simulink model "PubIfDecisionLSM_MDL"  (R2020b)
settings: configuration reference "DspaceConfig" (kept outside this file)
PostLoadFcn:
  | if any(exist('dsrtsu_mdlpostloadfcn', 'file') ~= 0), dsrtsu_mdlpostloadfcn('Execute', bdroot); end
InitFcn:
  | , if any(exist('rtifpga_mdlclblib', 'file') ~= 0), rtifpga_mdlclblib('Init', bdroot); end,
  | , if any(exist('dsmpb_private', 'file') ~= 0), dsmpb_private('dsmpb_mdlclblib', 'Init', bdroot); end,
values from neighbouring files (symbols this model uses):
  P_LSM_ALC_Enable = 0.0    [LSM_Parameter.sldd]
  P_LSM_AwayEdge_offset = 0.1    [LSM_Parameter.sldd]
  P_LSM_CentValidErr = 1.0    [LSM_Parameter.sldd]
  P_LSM_DOP_C0_EN_Limit = 0.8    [LSM_Parameter.sldd]
  P_LSM_DOP_C0_out_Limit = 2.0    [LSM_Parameter.sldd]
  P_LSM_DOP_C1_EN_Limit : value not decoded    [LSM_Parameter.sldd]
  P_LSM_DOP_C1_out_Limit : value not decoded    [LSM_Parameter.sldd]
  P_LSM_DOP_C1AndC2_Lim_X : value not decoded    [LSM_Parameter.sldd]
  P_LSM_DOP_C2_EN_Limit : value not decoded    [LSM_Parameter.sldd]
  P_LSM_DOP_C2_out_Limit : value not decoded    [LSM_Parameter.sldd]
  P_LSM_DOP_In_Pre2Dop_Dis = 1.0    [LSM_Parameter.sldd]
  P_LSM_DOP_Out_Pre2Dop_Dis = 2.0    [LSM_Parameter.sldd]
  P_LSM_DOP_PreDis_X : value not decoded    [LSM_Parameter.sldd]
  P_LSM_DOP_PreDis_Y : value not decoded    [LSM_Parameter.sldd]
  P_LSM_DOPEnableSW = 1.0    [LSM_Parameter.sldd]
  P_LSM_DOPValid_CheckTime = 0.06    [LSM_Parameter.sldd]
  P_LSM_DoubleLine_Curr2Cent_Dislimit = 0.5    [LSM_Parameter.sldd]
  P_LSM_DoubleLine_Dop2Cent_Dislimit = 0.5    [LSM_Parameter.sldd]
  P_LSM_DoubleLine_DOPOut_C1 : value not decoded    [LSM_Parameter.sldd]
  P_LSM_DoubleLine_Pre2Cent_Dislimit = 1.0    [LSM_Parameter.sldd]
  P_LSM_Error_Limit = 0.5    [LSM_Parameter.sldd]
  P_LSM_IFV2CenterAxis = 0.0    [LSM_Parameter.sldd]
  P_LSM_IFV2RearAxis = 0.0    [LSM_Parameter.sldd]
  P_LSM_Line2Edge_limit = 0.5    [LSM_Parameter.sldd]
  P_LSM_Line_Error = 0.1    [LSM_Parameter.sldd]
  P_LSM_LineSTD_Limit = 0.15    [LSM_Parameter.sldd]
  P_LSM_NOH_Switch = 0.0    [LSM_Parameter.sldd]
  P_LSM_OTL_C0_Factor = 1.0    [LSM_Parameter.sldd]
  P_LSM_OTL_C1_Factor = 0.5    [LSM_Parameter.sldd]
  P_LSM_OTL_C2_Factor = 0.5    [LSM_Parameter.sldd]
  P_LSM_Pre2OnlyLineDis = 5.0    [LSM_Parameter.sldd]
  P_LSM_Pre_t = 0.0    [LSM_Parameter.sldd]
  P_LSM_SingleLine_Cent2Edge_Dislimit = 100.0    [LSM_Parameter.sldd]
  P_LSM_SingleLine_Curr2Cent_Dislimit = 0.2    [LSM_Parameter.sldd]
  P_LSM_SingleLine_Dop2Cent_Dislimit = 0.2    [LSM_Parameter.sldd]
  P_LSM_SingleLine_DOPOut_C1 : value not decoded    [LSM_Parameter.sldd]
  P_LSM_SingleLine_Pre2Cent_Dislimit = 0.5    [LSM_Parameter.sldd]
  P_LSM_TJALimitSpd = 60.0    [LSM_Parameter.sldd]
undefined symbols (not defined in the file or in its folder): P_lCS_IFV2CenterAxis, P_LCS_IFV2RearAxis, P_LSM_EntryEdge_offset, P_LSM_EntryLnChngEnSwitch, P_LSM_EntryVanishDis, P_LSM_LinetLostTime, P_LSM_LineWijCal_C12, P_LSM_LineWijCal_C13, P_LSM_MapValid_ErrorSwitch, P_LSM_PosLineLcFac, P_LSM_SpdLim_Stub_Spd, P_LSM_SpdLim_StubLength, P_LSM_SpdTurnAlarm
libraries: simulink x324, TrueDurationTime x11
(part 20 of 25)

== matlab function PubIfDecisionLSM_MDL/Subsystem1/TargetLineCalc_20ms2/TargetLineCalc/HWALineCalc ==
  data: LeftLineTypeEn input boolean size=1; RightLineTypeEn input boolean size=1; YBranch_b input boolean size=1; YBranchRi_b input boolean size=1; HWALineC0K1 input; TJA_Line_State input; HWALineValid output boolean size=1; HWASts input uint8 size=1; HWAStsK1 input uint8 size=1; LineConf input uint8 size=4; Reliable input; A3 input single size=4; A2 input single size=4; A1 input single size=4; A0 input single size=4; Range input single size=4; tLost input single size=4; PathPredValid input boolean size=1; PathPredA3 input single size=1; PathPredA2 input single size=1; PathPredA1 input single size=1; PathPredA0 input single size=1; PathPredRange input; LeftOffset_b input boolean size=1; RightOffset_b input boolean size=1; HWALineC3 output single size=1; HWALineC2 output single size=1; HWALineC1 output single size=1; HWALineC0 output single size=1; HWARange output single size=1; RoadWidth input single size=1; dDeltaX input single size=1; dDeltaY input single size=1; CosOfPsi input single size=1; SinOfPsi input single size=1; vRef input single size=1; DistanceLim input single size=1; HWALeLineValid output boolean size=1; HWALeLineC3 output single size=1; HWALeLineC2 output single size=1; HWALeLineC1 output single size=1; HWALeLineC0 output single size=1; HWALeRange output single size=1; HWARiLineValid output boolean size=1; HWARiLineC3 output single size=1; HWARiLineC2 output single size=1; HWARiLineC1 output single size=1; HWARiLineC0 output single size=1; HWARiRange output single size=1; preDyDiff output single size=1; HeadAngDiff output single size=1; Error output boolean size=1; SingleLineLost_b output boolean size=1; DoubleLineLost_b output boolean size=1; MoveIDK1 input int8 size=1; LockIDK1 input int8; MoveID output int8 size=1; LockID output int8; Lock_counterK1 input uint8; Lock_counter output uint8
function [HWALineValid,HWALineC3,HWALineC2,HWALineC1,HWALineC0,HWARange,...
    HWALeLineValid,HWALeLineC3,HWALeLineC2,HWALeLineC1,HWALeLineC0,HWALeRange,...
    HWARiLineValid,HWARiLineC3,HWARiLineC2,HWARiLineC1,HWARiLineC0,HWARiRange,...
    preDyDiff,HeadAngDiff,Error,SingleLineLost_b,DoubleLineLost_b,MoveID,LockID,Lock_counter] = ...
    LineCalc(LeftLineTypeEn,RightLineTypeEn,YBranch_b,YBranchRi_b,HWALineC0K1,TJA_Line_State,HWASts,HWAStsK1,LineConf,Reliable,A3,A2,A1,A0,Range,tLost,...
    PathPredValid,PathPredA3,PathPredA2,PathPredA1,PathPredA0,PathPredRange,...
    LeftOffset_b,RightOffset_b,RoadWidth,dDeltaX,dDeltaY,CosOfPsi,SinOfPsi,vRef,DistanceLim,MoveIDK1,LockIDK1,Lock_counterK1)

HWALineValid = false;
HWALineC3 = single(0);
HWALineC2 = single(0);
HWALineC1 = single(0);
HWALineC0 = single(0);
HWARange = single(0);
HWALeLineValid = false;
HWALeLineC3 = single(0);
HWALeLineC2 = single(0);
HWALeLineC1 = single(0);
HWALeLineC0 = single(0);
HWALeRange = single(0);
HWARiLineValid = false;
HWARiLineC3 = single(0);
HWARiLineC2 = single(0);
HWARiLineC1 = single(0);
HWARiLineC0 = single(0);
HWARiRange = single(0);
Error = false;
SingleLineLost_b = false;
DoubleLineLost_b = false;
preDis = single(50);

MoveID = MoveIDK1;
LockID = LockIDK1;
if abs(HWALineC0K1)>4.5
    MoveID = int8(0);
    LockID = int8(0);
end

Lock_counter = max(Lock_counterK1-uint8(1),uint8(0));
if Lock_counter==0
    LockID = int8(0);
end

if (HWASts==1)||(HWASts==7)||(HWASts==0)
    MoveID = int8(0);
end

if HWASts ==1 || HWASts == 2
    HWALineValid = PathPredValid;
    HWALineC3 = PathPredA3;
    HWALineC2 = PathPredA2;
    HWALineC1 = PathPredA1;
    HWALineC0 = PathPredA0;
    HWARange = PathPredRange;
end
if HWASts==3 || HWASts==11 || HWASts==12
    MoveID = int8(0);
    if HWAStsK1==5 || HWAStsK1==6
        Lock_counter = uint8(250);
        LockID = int8(0);
    end
    if Lock_counter>0
        if LeftOffset_b
            LockID = LockID + int8(1);
        end
        if RightOffset_b
            LockID = LockID - int8(1);
        end
        if (LineConf(2+LockID)>0)&&(LineConf(3+LockID)>0)&&...
                max(Range(2+LockID),Range(3+LockID))>DistanceLim&&...
                ((tLost(2+LockID)<0.15)||(tLost(3+LockID)<0.15))
            if YBranch_b
                HWALineValid = true;
                HWALineC3 = A3(2+LockID);
                HWALineC2 = A2(2+LockID);
                HWALineC1 = A1(2+LockID);
                HWALineC0 = A0(2+LockID) - 0.5*RoadWidth*sqrt(single(1) + A1(2+LockID)*A1(2+LockID));
                HWARange = Range(2+LockID);
            else
                if Reliable(2+LockID)>0.5&&Reliable(3+LockID)>0.5
                    HWALineValid = true;
                    HWALineC3 = 0.5*(A3(2+LockID) + A3(3+LockID));
                    HWALineC2 = 0.5*(A2(2+LockID) + A2(3+LockID));
                    HWALineC1 = 0.5*(A1(2+LockID) + A1(3+LockID));
                    HWALineC0 = 0.5*(A0(2+LockID) + A0(3+LockID));
                    HWARange = max(Range(2+LockID),Range(3+LockID));
                elseif Reliable(2+LockID)>0.5
                    HWALineValid = true;
                    HWALineC3 = A3(2+LockID);
                    HWALineC2 = A2(2+LockID);
                    HWALineC1 = A1(2+LockID);
                    HWALineC0 = A0(2+LockID) - 0.5*RoadWidth*sqrt(single(1) + A1(2+LockID)*A1(2+LockID));
                    HWARange = Range(2+LockID);
                elseif Reliable(3+LockID)>0.5
                    HWALineValid = true;
                    HWALineC3 = A3(3+LockID);
                    HWALineC2 = A2(3+LockID);
                    HWALineC1 = A1(3+LockID);
                    HWALineC0 = A0(3+LockID) + 0.5*RoadWidth*sqrt(single(1) + A1(3+LockID)*A1(3+LockID));
                    HWARange = Range(3+LockID);
                end
            end
        elseif (LineConf(2+LockID)>0)&&...
                (Range(2+LockID)>DistanceLim)
            HWALineValid = true;
            HWALineC3 = A3(2+LockID);
            HWALineC2 = A2(2+LockID);
            HWALineC1 = A1(2+LockID);
            HWALineC0 = A0(2+LockID) - 0.5*RoadWidth*sqrt(single(1) + A1(2+LockID)*A1(2+LockID));
            HWARange = Range(2+LockID);
            if YBranch_b==false
                SingleLineLost_b = true;
            end
        elseif (LineConf(3+LockID)>0)&&...
                (Range(3+LockID)>DistanceLim)
            HWALineValid = true;
            HWALineC3 = A3(3+LockID);
            HWALineC2 = A2(3+LockID);
            HWALineC1 = A1(3+LockID);
            HWALineC0 = A0(3+LockID) + 0.5*RoadWidth*sqrt(single(1) + A1(3+LockID)*A1(3+LockID));
            HWARange = Range(3+LockID);
            SingleLineLost_b = true;
        else
            DoubleLineLost_b = true;
        end
    else
        LockID = int8(0);
        HWALineValid = PathPredValid;
        HWALineC3 = PathPredA3;
        HWALineC2 = PathPredA2;
        HWALineC1 = PathPredA1;
        HWALineC0 = PathPredA0;
        HWARange = PathPredRange;
    end
    
    if (LineConf(2)>0)&&(LineConf(1)>0)&&...
            (Range(2)>DistanceLim)&&(Range(1)>0.8*DistanceLim)&&...
            ((tLost(2)<0.15)||(tLost(1)<0.15))&&abs(A0(1)-A0(2))>3&&...
            abs(A0(1)+A1(1)*preDis+A2(1)*preDis^2+A3(1)*preDis^3-A0(2)-A1(2)*preDis-A2(2)*preDis^2-A3(2)*preDis^3)>3&&...
            TJA_Line_State==1
%             (LeftLineTypeEn)&&

        HWALeLineValid = true;
        HWALeLineC3 = 0.5*(A3(2) + A3(1));
        HWALeLineC2 = 0.5*(A2(2) + A2(1));
        HWALeLineC1 = 0.5*(A1(2) + A1(1));
        HWALeLineC0 = 0.5*(A0(2) + A0(1));
        if abs(HWALeLineC0)>4.5
            HWALeLineValid = false;
        end
        HWALeRange = 0.5*(Range(2) + Range(1));
    end
    if (LineConf(4)>0)&&(LineConf(3)>0)&&...
            (Range(4)>0.8*DistanceLim)&&(Range(3)>DistanceLim)&&...
            ((tLost(4)<0.15)||(tLost(3)<0.15))&&abs(A0(3)-A0(4))>3&&...
            abs(A0(3)+A1(3)*preDis+A2(3)*preDis^2+A3(3)*preDis^3-A0(4)-A1(4)*preDis-A2(4)*preDis^2-A3(4)*preDis^3)>3&&...
            TJA_Line_State==1
%             (RightLineTypeEn)
        HWARiLineValid = true;
        HWARiLineC3 = 0.5*(A3(4) + A3(3));
        HWARiLineC2 = 0.5*(A2(4) + A2(3));
        HWARiLineC1 = 0.5*(A1(4) + A1(3));
        HWARiLineC0 = 0.5*(A0(4) + A0(3));
        if abs(HWARiLineC0)>4.5
            HWARiLineValid = false;
        end
        HWARiRange = 0.5*(Range(4) + Range(3));
    end
end
if HWASts==5
    if HWAStsK1~=5
        MoveID = MoveID - int8(1);
    end
    if LeftOffset_b
        MoveID = MoveID + int8(1);
    end
    if RightOffset_b
        MoveID = MoveID - int8(1);
    end
    %     if MoveID==-1 && LeftLineTypeEn==0
    %         MoveID = int8(1);
    %     end
    if (MoveID>=1)||(MoveID<=-2)
        Error = true;
    end
    if Error==false
        if (LineConf(int8(2)+MoveID)>0)&&(LineConf(int8(3)+MoveID)>0)&&...
                (Range(int8(2)+MoveID)>0.8*DistanceLim)&&(Range(int8(3)+MoveID)>0.8*DistanceLim)&&...
                ((tLost(int8(2)+MoveID)<0.15)||(tLost(int8(3)+MoveID)<0.15))
            if MoveID~=0
%                 if LeftLineTypeEn==1
                    HWALineValid = true;
                    HWALineC3 = A3(int8(3)+MoveID);
                    HWALineC2 = A2(int8(3)+MoveID);
                    HWALineC1 = A1(int8(3)+MoveID);
                    HWALineC0 = A0(int8(3)+MoveID)+ 0.5*RoadWidth*sqrt(single(1) + A1(int8(3)+MoveID)*A1(int8(3)+MoveID));
                    HWARange = 0.5*(Range(int8(2)+MoveID) + Range(int8(3)+MoveID));
                    
                    HWALeLineValid = true;
                    HWALeLineC3 = A3(int8(3)+MoveID);
                    HWALeLineC2 = A2(int8(3)+MoveID);
                    HWALeLineC1 = A1(int8(3)+MoveID);
                    HWALeLineC0 = A0(int8(3)+MoveID)+ 0.5*RoadWidth*sqrt(single(1) + A1(int8(3)+MoveID)*A1(int8(3)+MoveID));
                    HWALeRange = 0.5*(Range(int8(2)+MoveID) + Range(int8(3)+MoveID));
%                 else
%                     HWALineValid = true;
%                     HWALineC3 = 0.5*(A3(int8(2)+MoveID) + A3(int8(3)+MoveID));
%                     HWALineC2 = 0.5*(A2(int8(2)+MoveID) + A2(int8(3)+MoveID));
%                     HWALineC1 = 0.5*(A1(int8(2)+MoveID) + A1(int8(3)+MoveID));
%                     HWALineC0 = 0.5*(A0(int8(2)+MoveID) + A0(int8(3)+MoveID));
%                     HWARange = 0.5*(Range(int8(2)+MoveID) + Range(int8(3)+MoveID));
%                 end
            else
                HWALineValid = true;
                HWALineC3 = 0.5*(A3(int8(2)+MoveID) + A3(int8(3)+MoveID));
                HWALineC2 = 0.5*(A2(int8(2)+MoveID) + A2(int8(3)+MoveID));
                HWALineC1 = 0.5*(A1(int8(2)+MoveID) + A1(int8(3)+MoveID));
                HWALineC0 = 0.5*(A0(int8(2)+MoveID) + A0(int8(3)+MoveID));
                HWARange = 0.5*(Range(int8(2)+MoveID) + Range(int8(3)+MoveID));
                
                HWALeLineValid = true;
                HWALeLineC3 = 0.5*(A3(int8(2)+MoveID) + A3(int8(3)+MoveID));
                HWALeLineC2 = 0.5*(A2(int8(2)+MoveID) + A2(int8(3)+MoveID));
                HWALeLineC1 = 0.5*(A1(int8(2)+MoveID) + A1(int8(3)+MoveID));
                HWALeLineC0 = 0.5*(A0(int8(2)+MoveID) + A0(int8(3)+MoveID));
                HWALeRange = 0.5*(Range(int8(2)+MoveID) + Range(int8(3)+MoveID));
            end
        elseif (LineConf(int8(2)+MoveID)>0)&&...
                (Range(int8(2)+MoveID)>DistanceLim)
            HWALineValid = true;
            HWALineC3 = A3(int8(2)+MoveID);
            HWALineC2 = A2(int8(2)+MoveID);
            HWALineC1 = A1(int8(2)+MoveID);
            HWALineC0 = A0(int8(2)+MoveID) - 0.5*RoadWidth*sqrt(single(1) + A1(int8(2)+MoveID)*A1(int8(2)+MoveID));
            HWARange = Range(int8(2)+MoveID);
            %             SingleLineLost_b = true;
            HWALeLineValid = true;
            HWALeLineC3 = A3(int8(2)+MoveID);
            HWALeLineC2 = A2(int8(2)+MoveID);
            HWALeLineC1 = A1(int8(2)+MoveID);
            HWALeLineC0 = A0(int8(2)+MoveID) - 0.5*RoadWidth*sqrt(single(1) + A1(int8(2)+MoveID)*A1(int8(2)+MoveID));
            HWALeRange = Range(int8(2)+MoveID);
        elseif (LineConf(int8(3)+MoveID)>0)&&...
                (Range(int8(3)+MoveID)>DistanceLim)
            if MoveID==0
                HWALineValid = true;
                HWALineC3 = A3(int8(3)+MoveID);
                HWALineC2 = A2(int8(3)+MoveID);
                HWALineC1 = A1(int8(3)+MoveID);
                HWALineC0 = A0(int8(3)+MoveID) + 0.5*RoadWidth*sqrt(single(1) + A1(int8(3)+MoveID)*A1(int8(3)+MoveID));
                HWARange = Range(int8(3)+MoveID);
                %             SingleLineLost_b = true;
                HWALeLineValid = true;
                HWALeLineC3 = A3(int8(3)+MoveID);
                HWALeLineC2 = A2(int8(3)+MoveID);
                HWALeLineC1 = A1(int8(3)+MoveID);
                HWALeLineC0 = A0(int8(3)+MoveID) + 0.5*RoadWidth*sqrt(single(1) + A1(int8(3)+MoveID)*A1(int8(3)+MoveID));
                HWALeRange = Range(int8(3)+MoveID);
            else
%                 if LeftLineTypeEn==1
                    HWALineValid = true;
                    HWALineC3 = A3(int8(3)+MoveID);
                    HWALineC2 = A2(int8(3)+MoveID);
                    HWALineC1 = A1(int8(3)+MoveID);
                    HWALineC0 = A0(int8(3)+MoveID) + 0.5*RoadWidth*sqrt(single(1) + A1(int8(3)+MoveID)*A1(int8(3)+MoveID));
                    HWARange = Range(int8(3)+MoveID);
                    %             SingleLineLost_b = true;
                    HWALeLineValid = true;
                    HWALeLineC3 = A3(int8(3)+MoveID);
                    HWALeLineC2 = A2(int8(3)+MoveID);
                    HWALeLineC1 = A1(int8(3)+MoveID);
                    HWALeLineC0 = A0(int8(3)+MoveID) + 0.5*RoadWidth*sqrt(single(1) + A1(int8(3)+MoveID)*A1(int8(3)+MoveID));
                    HWALeRange = Range(int8(3)+MoveID);
%                 else
%                     HWALineValid = true;
%                     HWALineC3 = A3(int8(3)+MoveID);
%                     HWALineC2 = A2(int8(3)+MoveID);
%                     HWALineC1 = A1(int8(3)+MoveID);
%                     HWALineC0 = A0(int8(3)+MoveID) - 0.5*RoadWidth*sqrt(single(1) + A1(int8(3)+MoveID)*A1(int8(3)+MoveID));
%                     HWARange = Range(int8(3)+MoveID);
%                 end
            end
        else
            DoubleLineLost_b = true;
        end
        if (LineConf(4+MoveID)>0)&&(LineConf(int8(3)+MoveID)>0)&&...
                (Range(4+MoveID)>0.8*DistanceLim)&&(Range(int8(3)+MoveID)>0.8*DistanceLim)&&...
                ((tLost(4+MoveID)<0.15)||(tLost(int8(3)+MoveID)<0.15))
            HWARiLineValid = true;
            HWARiLineC3 = 0.5*(A3(4+MoveID) + A3(int8(3)+MoveID));
            HWARiLineC2 = 0.5*(A2(4+MoveID) + A2(int8(3)+MoveID));
            HWARiLineC1 = 0.5*(A1(4+MoveID) + A1(int8(3)+MoveID));
            HWARiLineC0 = 0.5*(A0(4+MoveID) + A0(int8(3)+MoveID));
            HWARiRange = 0.5*(Range(4+MoveID) + Range(int8(3)+MoveID));
        end
    end
end
if HWASts==6
    if HWAStsK1~=6
        MoveID = MoveID + int8(1);
    end
    if LeftOffset_b
        MoveID = MoveID + int8(1);
    end
    if RightOffset_b
        MoveID = MoveID - int8(1);
    end
    %     if MoveID==1 && RightLineTypeEn==0
    %         MoveID = int8(2);
    %     end
    if (MoveID>=2)||(MoveID<=-1)
        Error = true;
    end
    if Error==false
        if (LineConf(int8(2)+MoveID)>0)&&(LineConf(int8(3)+MoveID)>0)&&...
                (Range(int8(2)+MoveID)>0.8*DistanceLim)&&(Range(int8(3)+MoveID)>0.8*DistanceLim)&&...
                ((tLost(int8(2)+MoveID)<0.15)||(tLost(int8(3)+MoveID)<0.15))
            if MoveID==0
                if YBranch_b
                    HWALineValid = true;
                    HWALineC3 = A3(int8(2)+MoveID);
                    HWALineC2 = A2(int8(2)+MoveID);
                    HWALineC1 = A1(int8(2)+MoveID);
                    HWALineC0 = A0(int8(2)+MoveID) - 0.5*RoadWidth*sqrt(single(1) + A1(int8(2)+MoveID)*A1(int8(2)+MoveID));
                    HWARange = Range(int8(2)+MoveID);
                    
                    HWARiLineValid = HWALineValid;
                    HWARiLineC3 = HWALineC3;
                    HWARiLineC2 = HWALineC2;
                    HWARiLineC1 = HWALineC1;
                    HWARiLineC0 = HWALineC0;
                    HWARiRange = HWARange;
                else
                    HWALineValid = true;
                    HWALineC3 = 0.5*(A3(int8(2)+MoveID) + A3(int8(3)+MoveID));
                    HWALineC2 = 0.5*(A2(int8(2)+MoveID) + A2(int8(3)+MoveID));
                    HWALineC1 = 0.5*(A1(int8(2)+MoveID) + A1(int8(3)+MoveID));
                    HWALineC0 = 0.5*(A0(int8(2)+MoveID) + A0(int8(3)+MoveID));
                    HWARange = 0.5*(Range(int8(2)+MoveID) + Range(int8(3)+MoveID));
                    
                    HWARiLineValid = HWALineValid;
                    HWARiLineC3 = HWALineC3;
                    HWARiLineC2 = HWALineC2;
                    HWARiLineC1 = HWALineC1;
                    HWARiLineC0 = HWALineC0;
                    HWARiRange = HWARange;
                end
            else
%                 if RightLineTypeEn==1
                    HWALineValid = true;
                    HWALineC3 = A3(int8(2)+MoveID);
                    HWALineC2 = A2(int8(2)+MoveID);
                    HWALineC1 = A1(int8(2)+MoveID);
                    HWALineC0 = A0(int8(2)+MoveID) - 0.5*RoadWidth*sqrt(single(1) + A1(int8(2)+MoveID)*A1(int8(2)+MoveID));
                    HWARange = Range(int8(2)+MoveID);
                    
                    HWARiLineValid = true;
                    HWARiLineC3 = A3(int8(2)+MoveID);
                    HWARiLineC2 = A2(int8(2)+MoveID);
                    HWARiLineC1 = A1(int8(2)+MoveID);
                    HWARiLineC0 = A0(int8(2)+MoveID) - 0.5*RoadWidth*sqrt(single(1) + A1(int8(2)+MoveID)*A1(int8(2)+MoveID));
                    HWARiRange = 0.5*(Range(int8(2)+MoveID) + Range(int8(3)+MoveID));
%                 else
%                     HWALineValid = true;
%                     HWALineC3 = 0.5*(A3(int8(2)+MoveID) + A3(int8(3)+MoveID));
%                     HWALineC2 = 0.5*(A2(int8(2)+MoveID) + A2(int8(3)+MoveID));
%                     HWALineC1 = 0.5*(A1(int8(2)+MoveID) + A1(int8(3)+MoveID));
%                     HWALineC0 = 0.5*(A0(int8(2)+MoveID) + A0(int8(3)+MoveID));
%                     HWARange = 0.5*(Range(int8(2)+MoveID) + Range(int8(3)+MoveID));
%                 end
            end
        elseif (LineConf(int8(2)+MoveID)>0)&&...
                (Range(int8(2)+MoveID)>DistanceLim)
            if MoveID==0
                HWALineValid = true;
                HWALineC3 = A3(int8(2)+MoveID);
                HWALineC2 = A2(int8(2)+MoveID);
                HWALineC1 = A1(int8(2)+MoveID);
                HWALineC0 = A0(int8(2)+MoveID) - 0.5*RoadWidth*sqrt(single(1) + A1(int8(2)+MoveID)*A1(int8(2)+MoveID));
                HWARange = Range(int8(2)+MoveID);
                %             SingleLineLost_b = true;
                HWARiLineValid = true;
                HWARiLineC3 = A3(int8(2)+MoveID);
                HWARiLineC2 = A2(int8(2)+MoveID);
                HWARiLineC1 = A1(int8(2)+MoveID);
                HWARiLineC0 = A0(int8(2)+MoveID) - 0.5*RoadWidth*sqrt(single(1) + A1(int8(2)+MoveID)*A1(int8(2)+MoveID));
                HWARiRange = Range(int8(2)+MoveID);
            else
%                 if RightLineTypeEn==1
                    HWALineValid = true;
                    HWALineC3 = A3(int8(2)+MoveID);
                    HWALineC2 = A2(int8(2)+MoveID);
                    HWALineC1 = A1(int8(2)+MoveID);
                    HWALineC0 = A0(int8(2)+MoveID) - 0.5*RoadWidth*sqrt(single(1) + A1(int8(2)+MoveID)*A1(int8(2)+MoveID));
                    HWARange = Range(int8(2)+MoveID);
                    %             SingleLineLost_b = true;
                    HWARiLineValid = true;
                    HWARiLineC3 = A3(int8(2)+MoveID);
                    HWARiLineC2 = A2(int8(2)+MoveID);
                    HWARiLineC1 = A1(int8(2)+MoveID);
                    HWARiLineC0 = A0(int8(2)+MoveID) - 0.5*RoadWidth*sqrt(single(1) + A1(int8(2)+MoveID)*A1(int8(2)+MoveID));
                    HWARiRange = Range(int8(2)+MoveID);
%                 else
%                     HWALineValid = true;
%                     HWALineC3 = A3(int8(2)+MoveID);
%                     HWALineC2 = A2(int8(2)+MoveID);
%                     HWALineC1 = A1(int8(2)+MoveID);
%                     HWALineC0 = A0(int8(2)+MoveID) - 0.5*RoadWidth*sqrt(single(1) + A1(int8(2)+MoveID)*A1(int8(2)+MoveID));
%                     HWARange = Range(int8(2)+MoveID);
%                 end
            end
        elseif (LineConf(int8(3)+MoveID)>0)&&...
                (Range(int8(3)+MoveID)>DistanceLim)
            HWALineValid = true;
            HWALineC3 = A3(int8(3)+MoveID);
            HWALineC2 = A2(int8(3)+MoveID);
            HWALineC1 = A1(int8(3)+MoveID);
            HWALineC0 = A0(int8(3)+MoveID) + 0.5*RoadWidth*sqrt(single(1) + A1(int8(3)+MoveID)*A1(int8(3)+MoveID));
            HWARange = Range(int8(3)+MoveID);
            %             SingleLineLost_b = true;
            HWARiLineValid = true;
            HWARiLineC3 = A3(int8(3)+MoveID);
            HWARiLineC2 = A2(int8(3)+MoveID);
            HWARiLineC1 = A1(int8(3)+MoveID);
            HWARiLineC0 = A0(int8(3)+MoveID) + 0.5*RoadWidth*sqrt(single(1) + A1(int8(3)+MoveID)*A1(int8(3)+MoveID));
            HWARiRange = Range(int8(3)+MoveID);
        else
            DoubleLineLost_b = true;
        end
        if (LineConf(1+MoveID)>0)&&(LineConf(int8(2)+MoveID)>0)&&...
                (Range(1+MoveID)>0.8*DistanceLim)&&(Range(int8(2)+MoveID)>0.8*DistanceLim)&&...
                ((tLost(1+MoveID)<0.15)||(tLost(int8(2)+MoveID)<0.15))
            HWALeLineValid = true;
            HWALeLineC3 = 0.5*(A3(1+MoveID) + A3(int8(2)+MoveID));
            HWALeLineC2 = 0.5*(A2(1+MoveID) + A2(int8(2)+MoveID));
            HWALeLineC1 = 0.5*(A1(1+MoveID) + A1(int8(2)+MoveID));
            HWALeLineC0 = 0.5*(A0(1+MoveID) + A0(int8(2)+MoveID));
            HWALeRange = 0.5*(Range(1+MoveID) + Range(int8(2)+MoveID));
        end
    end
end

%% SafeStop  slowExit
if (HWASts==9)||(HWASts==10)
    %     if (HWAStsK1~=9)&&(HWAStsK1~=10)
    %         MoveID = int8(0);
    %     else
    if LeftOffset_b
        LockID = LockID + int8(1);
    end
    if RightOffset_b
        LockID = LockID - int8(1);
    end
    %     end
    if (LineConf(int8(2)+LockID)>0)&&(LineConf(int8(3)+LockID)>0)&&...
            (Range(int8(2)+LockID)>0.5*DistanceLim)&&(Range(int8(3)+LockID)>0.5*DistanceLim)
        HWALineValid = true;
        HWALineC3 = 0.5*(A3(int8(2)+LockID) + A3(int8(3)+LockID));
        HWALineC2 = 0.5*(A2(int8(2)+LockID) + A2(int8(3)+LockID));
        HWALineC1 = 0.5*(A1(int8(2)+LockID) + A1(int8(3)+LockID));
        HWALineC0 = 0.5*(A0(int8(2)+LockID) + A0(int8(3)+LockID));
        HWARange = 0.5*(Range(int8(2)+LockID) + Range(int8(3)+LockID));
    elseif (LineConf(int8(2)+LockID)>0)&&...
            (Range(int8(2)+LockID)>0.5*DistanceLim)
        HWALineValid = true;
        HWALineC3 = A3(int8(2)+LockID);
        HWALineC2 = A2(int8(2)+LockID);
        HWALineC1 = A1(int8(2)+LockID);
        HWALineC0 = A0(int8(2)+LockID) - 0.5*RoadWidth*sqrt(single(1) + A1(int8(2)+LockID)*A1(int8(2)+LockID));
        HWARange = Range(int8(2)+LockID);
        SingleLineLost_b = true;
    elseif (LineConf(int8(3)+LockID)>0)&&...
            (Range(int8(3)+LockID)>0.5*DistanceLim)
        HWALineValid = true;
        HWALineC3 = A3(int8(3)+LockID);
        HWALineC2 = A2(int8(3)+LockID);
        HWALineC1 = A1(int8(3)+LockID);
        HWALineC0 = A0(int8(3)+LockID) + 0.5*RoadWidth*sqrt(single(1) + A1(int8(3)+LockID)*A1(int8(3)+LockID));
        HWARange = Range(int8(3)+LockID);
        SingleLineLost_b = true;
    else
        DoubleLineLost_b = true;
    end
end

%% Double Line Lost
if DoubleLineLost_b==true
    if ((HWASts==3)||(HWASts==4)||(HWASts==5)||(HWASts==6)||(HWASts==9))
        HWALineValid = PathPredValid;
        HWALineC3 = PathPredA3;
        HWALineC2 = PathPredA2;
        HWALineC1 = PathPredA1;
        HWALineC0 = PathPredA0;
    end
end
t_Dist = max(single(15),vRef*1.8);
x = [0.05*t_Dist;0.3*t_Dist;0.6*t_Dist;t_Dist];
t_dx = x-dDeltaX;
Y_Tar = HWALineC3*x.^3 + HWALineC2*x.^2 + HWALineC1*x + HWALineC0;
dy_Tar = Y_Tar-dDeltaY;
TmpX = t_dx*CosOfPsi+dy_Tar*SinOfPsi;
TmpY = -t_dx*SinOfPsi+dy_Tar*CosOfPsi;
[~,~,HeadAng_Error,preDyDiff] = pl(TmpX,TmpY);
HeadAngDiff = atan(HeadAng_Error)*57.3;
% xOffset = single(2.1);
%
% t_dyDiff = HWALineA3*xOffset^3 + HWALineA2*xOffset^2 + HWALineA1*xOffset + HWALineA0;
% t_A1 = 3*HWALineA3*xOffset^2 + 2*HWALineA2*xOffset + HWALineA1;
% dyDiff = t_dyDiff/sqrt(single(1) + t_A1^2);

== matlab function PubIfDecisionLSM_MDL/Subsystem1/TargetLineCalc_20ms2/TargetLineCalc/LREWidthCalc ==
  data: LRELineConf input uint8 size=2; a1 input single size=2; a0 input single size=2; LRELineUpdate input boolean size=1; LREWidthK1 input single size=1; LREWidth output single size=1
function LREWidth  = VisRoadWidth(LRELineConf,a1,a0,LRELineUpdate,LREWidthK1)

LREWidth = LREWidthK1;
Update = false;
temp = single(0);

if LRELineUpdate
    if (LRELineConf(1)>0)&&(LRELineConf(2)>0)
        if abs(57.3*(atan(a1(1)) - atan(a1(2))))<3
            temp = (a0(1) - a0(2))/sqrt(a1(2)^2 + single(1));
            Update = true;
        end
    end
    if Update
        LREWidth = 0.1*(temp - LREWidthK1) + LREWidthK1;
    end
end

== matlab function PubIfDecisionLSM_MDL/Subsystem1/TargetLineCalc_20ms2/TargetLineCalc/LineSelect ==
  data: TJALineValid output boolean size=1; CentLaneValid input boolean size=1; CentLineA3 input single size=1; CentLineA2 input single size=1; CentLineA1 input single size=1; CentLineA0 input single size=1; CentRange input single size=1; OTLineValid input boolean size=1; aOTL input single size=1; bOTL input single size=1; cOTL input single size=1; dOTL input single size=1; dxMax input single size=1; TJA_Line_State input; TJALineA3 output single size=1; TJALineA2 output single size=1; TJALineA1 output single size=1; TJALineA0 output single size=1; TJALineRange output single size=1; LCKLineValid output boolean size=1; LCKLineA3 output single size=1; LCKLineA2 output single size=1; LCKLineA1 output single size=1; LCKLineA0 output single size=1; LCKLineRange output single size=1
function [TJALineValid,TJALineA3,TJALineA2,TJALineA1,TJALineA0,TJALineRange,...
    LCKLineValid,LCKLineA3,LCKLineA2,LCKLineA1,LCKLineA0,LCKLineRange] = ...
    LineSelect(CentLaneValid,CentLineA3,CentLineA2,CentLineA1,CentLineA0,CentRange,...
    OTLineValid,aOTL,bOTL,cOTL,dOTL,dxMax,TJA_Line_State)

TJALineValid = false;
TJALineA3 = single(0);
TJALineA2 = single(0);
TJALineA1 = single(0);
TJALineA0 = single(0);
TJALineRange = single(0);

if (CentLaneValid==true)&&(CentRange>12)
    LCKLineValid = true;
    LCKLineA3 = CentLineA3;
    LCKLineA2 = CentLineA2;
    LCKLineA1 = CentLineA1;
    LCKLineA0 = CentLineA0;
    LCKLineRange = CentRange;
else
    LCKLineValid = false;
    LCKLineA3 = single(0);
    LCKLineA2 = single(0);
    LCKLineA1 = single(0);
    LCKLineA0 = single(0);
    LCKLineRange = single(0);
end

% TJALimitSpd = 20;
% temp = (TJALimitSpd - 1.3)/1.03;
% temp = temp/3.6;


if TJA_Line_State == 1 || TJA_Line_State == 0
   
    TJALineValid = CentLaneValid;
    TJALineA3 = CentLineA3;
    TJALineA2 = CentLineA2;
    TJALineA1 = CentLineA1;
    TJALineA0 = CentLineA0;
    TJALineRange = CentRange;
elseif TJA_Line_State == 2
    TJALineValid = OTLineValid;
    TJALineA3 = aOTL;
    TJALineA2 = bOTL;
    TJALineA1 = cOTL;
    TJALineA0 = dOTL;
    TJALineRange = dxMax;
end

== matlab function PubIfDecisionLSM_MDL/Subsystem1/TargetLineCalc_20ms2/TargetLineCalc/MATLAB Function ==
  data: Cur_avail input; MrcStopLane output; Cur_LaneType input; Right_avail input
function MrcStopLane = fcn(Cur_avail,Cur_LaneType,Right_avail)
MrcStopLane = uint8(0);
if (Cur_avail>0&&Cur_LaneType==5)||(Cur_avail>0&&Cur_LaneType~=5&&Right_avail==0)
    MrcStopLane = uint8(1);
end

== matlab function PubIfDecisionLSM_MDL/Subsystem1/TargetLineCalc_20ms2/TargetLineCalc/MATLAB Function1 ==
  data: HWASts input uint8 size=1; HWALeLineValid output boolean size=1; RoadWidth input single size=1; LineValid input boolean size=1; LineC3 input single size=1; LineC2 input single size=1; LineC1 input single size=1; LineC0 input single size=1; LineRange input single size=1; LeLineValid input boolean size=1; LeLineC3 input single size=1; LeLineC2 input single size=1; LeLineC1 input single size=1; LeLineC0 input single size=1; LeLineRange input single size=1; RiLineValid input boolean size=1; RiLineC3 input single size=1; RiLineC2 input single size=1; RiLineC1 input single size=1; RiLineC0 input single size=1; RiLineRange input single size=1; HWALeLineC3 output single size=1; HWALeLineC2 output single size=1; HWALeLineC1 output single size=1; HWALeLineC0 output single size=1; HWALeLineRange output single size=1; LeLineVirtual_b output boolean size=1; HWARiLineValid output boolean size=1; HWARiLineC3 output single size=1; HWARiLineC2 output single size=1; HWARiLineC1 output single size=1; HWARiLineC0 output single size=1; HWARiLineRange output single size=1; RiLineVirtual_b output boolean size=1
function [HWALeLineValid,HWALeLineC3,HWALeLineC2,HWALeLineC1,HWALeLineC0,HWALeLineRange,LeLineVirtual_b,...
    HWARiLineValid,HWARiLineC3,HWARiLineC2,HWARiLineC1,HWARiLineC0,HWARiLineRange,RiLineVirtual_b]...
    = LineAddCalc(HWASts,RoadWidth,LineValid,LineC3,LineC2,LineC1,LineC0,LineRange,...
    LeLineValid,LeLineC3,LeLineC2,LeLineC1,LeLineC0,LeLineRange,...
    RiLineValid,RiLineC3,RiLineC2,RiLineC1,RiLineC0,RiLineRange)

if LeLineValid==true||HWASts~=3
    HWALeLineValid = LeLineValid;
    HWALeLineC3 = LeLineC3;
    HWALeLineC2 = LeLineC2;
    HWALeLineC1 = LeLineC1;
    HWALeLineC0 = LeLineC0;
    HWALeLineRange = LeLineRange;
    LeLineVirtual_b = false;
else
    HWALeLineValid = false;
    HWALeLineC3 = LineC3;
    HWALeLineC2 = LineC2;
    HWALeLineC1 = LineC1;
    HWALeLineC0 = LineC0 + RoadWidth;
    HWALeLineRange = LineRange;
    LeLineVirtual_b = true;
end

if RiLineValid==true||HWASts~=3
    HWARiLineValid = RiLineValid;
    HWARiLineC3 = RiLineC3;
    HWARiLineC2 = RiLineC2;
    HWARiLineC1 = RiLineC1;
    HWARiLineC0 = RiLineC0;
    HWARiLineRange = RiLineRange;
    RiLineVirtual_b = false;
else
    HWARiLineValid = false;
    HWARiLineC3 = LineC3;
    HWARiLineC2 = LineC2;
    HWARiLineC1 = LineC1;
    HWARiLineC0 = LineC0 - RoadWidth;
    HWARiLineRange = LineRange;
    RiLineVirtual_b = true;
end
